simulink model "nonlinear"  (R2017b)
settings: Solver=FixedStepAuto  StartTime=0.0  StopTime=100  FixedStep=10e-5
settings Model: Creator=Mehmet  LastModifiedBy=Mehmet

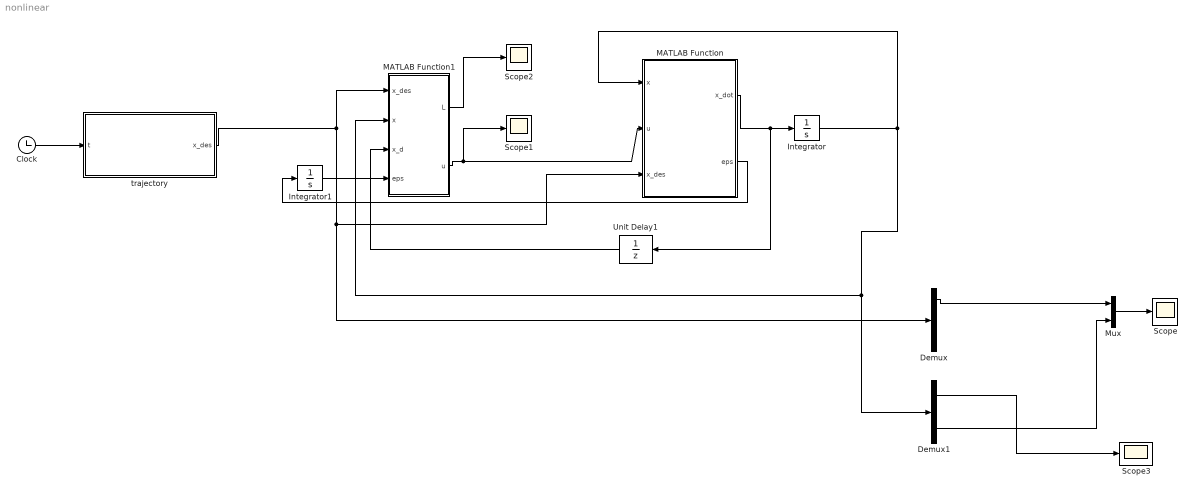
== system nonlinear ==
  Clock : Clock
  Demux : Demux  Outputs=3
  Demux1 : Demux  Outputs=2
  Integrator : Integrator  InitialCondition=[1;-1]
  Integrator1 : Integrator
  MATLAB Function : MATLAB Function  TreatAsAtomicUnit=on
  MATLAB Function1 : MATLAB Function  TreatAsAtomicUnit=on
  Mux : Mux  Inputs=2
  Scope{,1..3} (4 alike) : Scope
  Unit Delay1 : UnitDelay  InitialCondition=[0;0]  SampleTime=-1
  trajectory : MATLAB Function  TreatAsAtomicUnit=on
  wires:
  Clock/1 -> trajectory/1(t)
  trajectory/1(x_des) -> MATLAB Function1/1(x_des), MATLAB Function/3(x_des), Demux/1
  Mux/1 -> Scope/1
  MATLAB Function/1(x_dot) -> Unit Delay1/1, Integrator/1
  Integrator/1 -> Demux1/1, MATLAB Function1/2(x), MATLAB Function/1(x)
  MATLAB Function1/2(u) -> Scope1/1, MATLAB Function/2(u)
  MATLAB Function1/1(L) -> Scope2/1
  Demux/1 -> Mux/1
  Unit Delay1/1 -> MATLAB Function1/3(x_d)
  Demux1/1 -> Scope3/1
  Demux1/2 -> Mux/2
  Integrator1/1 -> MATLAB Function1/4(eps)
  MATLAB Function/2(eps) -> Integrator1/1

== matlab function nonlinear/MATLAB Function1 ==
  data: L output; x_des input; u output; x input; x_d input; eps input
function [L,u]= fcn(x_des,x,x_d,eps)

lam = 10;
Kv = 100;
Ki = 20;

e = x_des(1,1) - x(2,1);
e_d = x_des(2,1) - x_d(2,1);

r = e_d + lam*(e);

% system constant
A = -20;
B = 1;
C = 5.3;
D = 20;

zeta1 = C*A + cos(x(1))*A;
zeta2 = C*B + B*cos(x(1));
zeta3 = C + cos(x(1));


% define f(x) function
f_x = x_des(3) + lam*e_d - (zeta1*x(1) + zeta2*x(2)) - D*(x_des(2) + lam*e);

u = 1/zeta3*(f_x + Kv*r + Ki*eps);


L = 1/2*(e^2);

end

== matlab function nonlinear/MATLAB Function ==
  data: x input; u input; x_dot output; x_des input; eps output
function [x_dot,eps]= fcn(x,u,x_des)

q = zeros(2,1);

q(1,1) = -20*x(1,1) + 1*x(2,1) + u(1,1);
q(2,1) = 5.3*x(1,1) + 20*x(2,1) + sin(x(1,1));

x_dot = q;


eps = x_des(1) - x(2,1);

end

== matlab function nonlinear/trajectory ==
  data: t input; x_des output
function x_des = fcn(t)

% A = 10;
% B = 1;
% f = 0.11;
% w = 2*pi*f;
% 
% y = A*sin(w*t) + 20;
% y_d = A*w*cos(w*t);
% y_dd = -A*w*w*sin(w*t);

y = 0;

if t > 0 && t < 25
    
    y = 25 + t^2;
end

if t >= 25 && t < 50
    
    y = 35 - t^2;
    
end

if t >= 50 && t < 75
    
    y = 10 + t^2;
    
end

if t >= 75 && t < 100
    
    y = 20 - t^2;
    
end


y_d = 0;
y_dd = 0;


x_des = [y y_d y_dd]';

end
